simulink model "Temporal1"  (Simulink 5.0)
settings: Solver=ode45  StartTime=0.0  StopTime=10.0  RelTol=1e-3
settings Model: Creator=scaife  LastModifiedBy=scaife  ExtModeAutoUpdateStatusClock=off

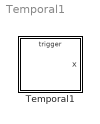
== system Temporal1 ==
  Temporal1 : Stateflow chart

== stateflow chart Temporal1 ==
  state A/
    x++;
  state B/
    x++;
  (default) -> A
  A -> B : E[after(2,E)]
  B -> A : after(3,E)
  data: x output int32
  events: E input RISING_EDGE_EVENT
